simulink model "fuzzyReg_v10"  (R2022b)
settings: Solver=ode45  StartTime=0.0  StopTime=4  RelTol=1e-6  EnableMultiTasking=on
model workspace (MAT data in the model file):
  fuzzy33_v2 : mamfis (value not decoded)
  fuzzy55 : mamfis (value not decoded)
  fuzzy55_v2 : mamfis (value not decoded)
undefined symbols (not defined in the file or in its folder): Cfi, Imax, J, Jc, Ka, KI, KR, KRw, KTM, Kw, Mz, sigbuilder_block, Ta, TI, TIw, TTM, Un, w0
libraries: fuzblock x4
settings Model: Creator=Samuel  LastModifiedBy=hwswi
settings SolverCC: AlgebraicLoopSolver=TrustRegion
settings DataIOCC: LimitDataPoints=on  SaveFormat=Array  ReturnWorkspaceOutputs=off
settings OptimizationCC: LifeSpan=inf
settings DebuggingCC: UnconnectedInputMsg=warning  UnconnectedOutputMsg=warning  UnconnectedLineMsg=warning  SFUnexpectedBacktrackingDiag=warning  SFNoUnconditionalDefaultTransitionDiag=warning  SFExecutionAtInitializationDiag=none  SFMachineParentedDataDiag=warning  ArithmeticOperatorsInVariantConditions=warning
settings HardwareCC: ProdBitPerPointer=32  ProdBitPerSizeT=32  ProdBitPerPtrDiffT=32  ProdLargestAtomicFloat=None  ProdIntDivRoundTo=Undefined  ProdEndianess=Unspecified  ProdWordSize=32  ProdHWDeviceType=32-bit Generic
settings ModelReferenceCC: PropagateSignalLabelsOutOfModel=off
settings SFSimCC: SimUseLocalCustomCode=off  CustomCodeUndefinedFunction=UseInterfaceOnly
settings RTWCC: RTWUseLocalCustomCode=off
settings CodeAppCC: StateflowObjectComments=on
settings GRTTargetCC: TargetLangStandard=C89/C90 (ANSI)
settings ConfigComp: CovMetricSettings=dw  CovSaveCumulativeToWorkspaceVar=on  CovSaveSingleToWorkspaceVar=on  CovExternalEMLEnable=off

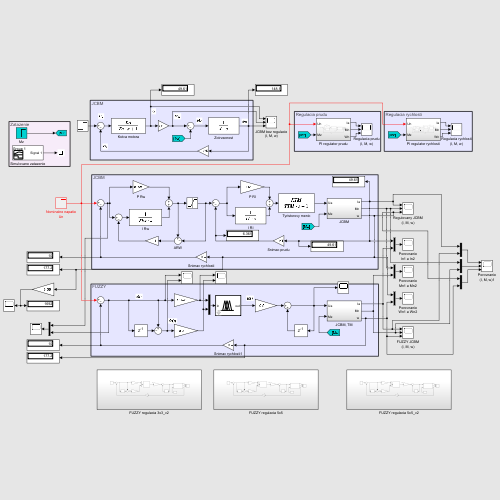
[thumbnail: Simulink's stored preview of the top-level diagram]
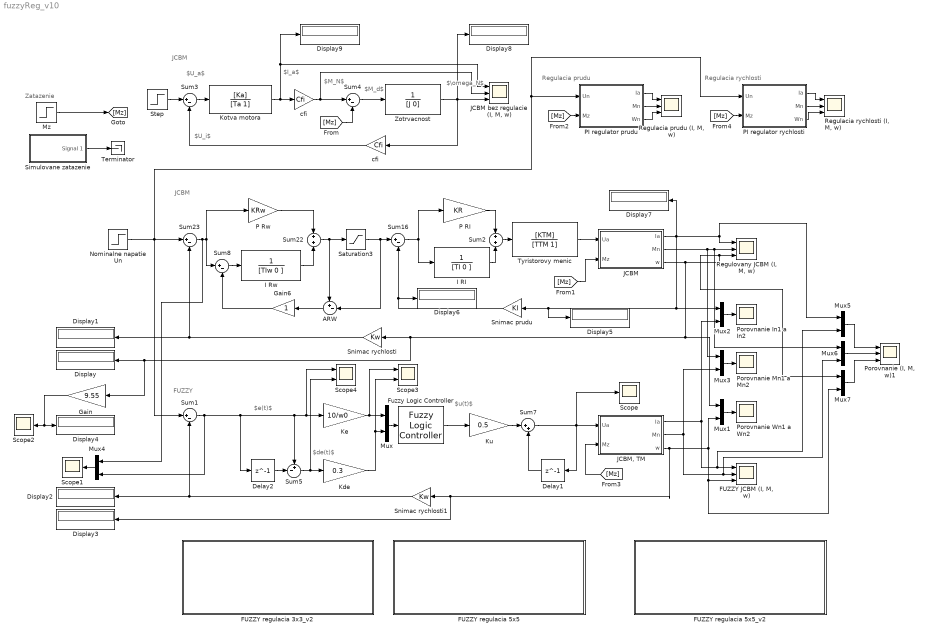
== system fuzzyReg_v10 ==
  note: Regulacia prudu
  note: Zatazenie
  note: JCBM
  note: FUZZY
  note: JCBM
  note: $M_N$
  note: $M_d$
  note: $I_a$
  note: $U_a$
  note: $U_i$
  note: $\omega_N$
  note: $e(t)$
  note: $de(t)$
  note: $u(t)$
  note: Regulacia rychlosti
  ARW : Sum  Inputs=+-|
  Delay1 : Delay  DelayLength=1  InitialCondition=0  SampleTime=0.018
  Delay2 : Delay  DelayLength=1  InitialCondition=0  SampleTime=0.018
  Display{,1..9} (10 alike) : Display
  "FUZZY JCBM (I, M, w)" : Scope  NumInputPorts=3
  FUZZY regulacia 3x3_v2 : Subsystem
  FUZZY regulacia 5x5 : Subsystem
  FUZZY regulacia 5x5_v2 : Subsystem
  Fuzzy Logic Controller : fuzblock/Fuzzy Logic  Controller  FIS=fuzzy55_v2  OutputSampleNumber=101  DataType=double  FuzzifiedInputs=off  RuleFiringStrengths=off  RuleOutputs=off  AggregatedOutputs=off  SimulateUsing=Interpreted execution  OutOfRangeInputValueMessage=warning  NoRuleFiredMessage=warning  EmptyOutputFuzzySetMessage=warning
  Gain : Gain  Gain=9.55
  Gain6 : Gain
  I RI : TransferFcn  Denominator=[TI 0 ]
  I Rw : TransferFcn  Denominator=[TIw 0 ]
  JCBM : Subsystem
  "JCBM bez regulacie (I, M, w)" : Scope  NumInputPorts=3
  "JCBM, TM" : Subsystem
  Kde : Gain  Gain=0.3
  Ke : Gain  Gain=10/w0
  Kotva motora : TransferFcn  Numerator=[Ka]  Denominator=[Ta 1]
  Ku : Gain  Gain=0.5
  Mux{,1..7} (8 alike) : Mux  Inputs=2
  Mz : Step  Time=2  After=Mz  SampleTime=0
  Nominalne napatie Un : Step  Time=0  After=10  SampleTime=0
  P RI : Gain  Gain=KR
  P Rw : Gain  Gain=KRw
  PI regulator prudu : Subsystem
  PI regulator rychlosti : Subsystem
  "Porovnanie (I, M, w)1" : Scope  NumInputPorts=3
  Porovnanie In1 a In2 : Scope
  Porovnanie Mn1 a Mn2 : Scope
  Porovnanie Wn1 a Wn2 : Scope
  "Regulacia prudu (I, M, w)" : Scope  NumInputPorts=3
  "Regulacia rychlosti (I, M, w)" : Scope  NumInputPorts=3
  "Regulovany JCBM (I, M, w)" : Scope  NumInputPorts=3
  Saturation3 : Saturate  UpperLimit=10  LowerLimit=-10
  Scope : Scope
  Scope1 : Scope
  Scope2 : Scope
  Scope3 : Scope  NumInputPorts=2
  Scope4 : Scope  NumInputPorts=2
  Simulovane zatazenie : Subsystem  Tag=STV Subsys  LoadFcn=sigbuilder_block('load');  StartFcn=sigbuilder_block('start');  StopFcn=sigbuilder_block('stop');  ClipboardFcn=sigbuilder_block('clipboard');  mask(Sigbuilder block){tuvar=[0:10]}
      mask help: Simulink:masks:SigbuilderBlock_MD
      mask init:
      | if ~strcmp(get_param(bdroot(gcbh),'SimulationStatus'),'stopped') tuvar = sigbuilder_block('maskInit'); end
      settings: CopyFcn=sigbuilder_block('copy');  DeleteFcn=sigbuilder_block('delete');  ModelCloseFcn=sigbuilder_block('modelClose');  PreSaveFcn=sigbuilder_block('preSave');  PauseFcn=sigbuilder_block('pause');  ContinueFcn=sigbuilder_block('continue');  NameChangeFcn=sigbuilder_block('namechange');  OpenFcn=sigbuilder_block('open',[717 162.75 551.25 360 ]);  CloseFcn=sigbuilder_block('close');
      mask Display: plot(0, 0, 100, 100,[2, 2, 32, 32, 2], [68, 8, 8, 68, 68],[32, 2], [38, 38], [32, 19, 2],[53, 60, 44], [32, 17, 17, 2],[16, 16, 31, 31]);txt = getActiveGroup(gcbh);text(2, 100, txt,'verticalAlignment', 'top');
  Snimac prudu : Gain  Gain=KI
  Snimac rychlosti : Gain  Gain=Kw
  Snimac rychlosti1 : Gain  Gain=Kw
  Step : Step  Time=0  After=Un  SampleTime=0
  Sum{1,3..4,8,16,23} (6 alike) : Sum  Inputs=|+-
  Sum2 : Sum
  Sum22 : Sum
  Sum5 : Sum  Inputs=+-|
  Sum7 : Sum  Inputs=|++
  Terminator : Terminator
  Tyristorovy menic : TransferFcn  Numerator=[KTM]  Denominator=[TTM 1]
  Zotrvacnost : TransferFcn  Denominator=[J 0]
  cfi : Gain  Gain=Cfi
  "cfi " : Gain  Gain=Cfi
  wires:
  Mux1/1 -> Porovnanie Wn1 a Wn2/1
  Mux2/1 -> Porovnanie In1 a In2/1
  Gain6/1 -> Sum8/2
  Sum8/1 -> I Rw/1
  ARW/1 -> Gain6/1
  Snimac rychlosti/1 -> Sum23/2, Display1/1
  Sum22/1 -> Saturation3/1, ARW/1
  I Rw/1 -> Sum22/2
  P Rw/1 -> Sum22/1
  Tyristorovy menic/1 -> JCBM/1(Ua)
  Sum23/1 -> Sum8/1, P Rw/1, Mux4/1
  Snimac prudu/1 -> Display6/1, Sum16/2
  Saturation3/1 -> ARW/2, Sum16/1
  Sum16/1 -> I RI/1, P RI/1
  Sum2/1 -> Tyristorovy menic/1
  I RI/1 -> Sum2/2
  P RI/1 -> Sum2/1
  JCBM/1(Ia) -> Display7/1, Mux5/1, "Regulovany JCBM (I, M, w)"/1, Mux2/1, Display5/1, Snimac prudu/1
  "JCBM, TM"/1(Ia) -> Mux2/2, Mux5/2, "FUZZY JCBM (I, M, w)"/1
  Sum5/1 -> Kde/1, Scope4/2
  Kde/1 -> Scope3/2, Mux/2
  Delay1/1 -> Sum7/2
  Delay2/1 -> Sum5/2
  Ke/1 -> Scope3/1, Mux/1
  Sum7/1 -> Delay1/1, Scope/1, "JCBM, TM"/1(Ua)
  Ku/1 -> Sum7/1
  Zotrvacnost/1 -> Display8/1, "JCBM bez regulacie (I, M, w)"/3, cfi/1
  cfi/1 -> Sum3/2
  Sum4/1 -> Zotrvacnost/1
  "cfi "/1 -> "JCBM bez regulacie (I, M, w)"/2, Sum4/1
  Sum3/1 -> Kotva motora/1
  [Mz] -> Sum4/2
  Mz/1 -> [Mz]
  [Mz] -> JCBM/2(Mz)
  PI regulator prudu/2(Mn) -> "Regulacia prudu (I, M, w)"/2
  PI regulator prudu/1(Ia) -> "Regulacia prudu (I, M, w)"/1
  PI regulator prudu/3(Wn) -> "Regulacia prudu (I, M, w)"/3
  [Mz] -> PI regulator prudu/2(Mz)
  "JCBM, TM"/2(" Mn ") -> Mux3/2, "FUZZY JCBM (I, M, w)"/2, Mux6/2
  JCBM/2(" Mn ") -> Mux3/1, "Regulovany JCBM (I, M, w)"/2, Mux6/1
  Mux3/1 -> Porovnanie Mn1 a Mn2/1
  Mux/1 -> Fuzzy Logic Controller/1
  Fuzzy Logic Controller/1 -> Ku/1
  [Mz] -> "JCBM, TM"/2(Mz)
  JCBM/3("w ") -> Mux7/1, "Regulovany JCBM (I, M, w)"/3, Mux1/1, Gain/1, Display/1, Snimac rychlosti/1
  Mux5/1 -> "Porovnanie (I, M, w)1"/1
  Mux6/1 -> "Porovnanie (I, M, w)1"/2
  Mux7/1 -> "Porovnanie (I, M, w)1"/3
  Snimac rychlosti1/1 -> Sum1/2, Display2/1
  Mux4/1 -> Scope1/1
  Gain/1 -> Scope2/1, Display4/1
  Sum1/1 -> Delay2/1, Ke/1, Scope4/1, Sum5/1, Mux4/2
  "JCBM, TM"/3("w ") -> Display3/1, Snimac rychlosti1/1, "FUZZY JCBM (I, M, w)"/3, Mux7/2, Mux1/2
  Nominalne napatie Un/1 -> Sum23/1, Sum1/1, PI regulator rychlosti/1(Un), PI regulator prudu/1(Un)
  Kotva motora/1 -> Display9/1, "JCBM bez regulacie (I, M, w)"/1, "cfi "/1
  Step/1 -> Sum3/1
  [Mz] -> PI regulator rychlosti/2(Mz)
  PI regulator rychlosti/3(Wn) -> "Regulacia rychlosti (I, M, w)"/3
  PI regulator rychlosti/1(Ia) -> "Regulacia rychlosti (I, M, w)"/1
  PI regulator rychlosti/2(Mn) -> "Regulacia rychlosti (I, M, w)"/2
  Simulovane zatazenie/1(Signal 1) -> Terminator/1

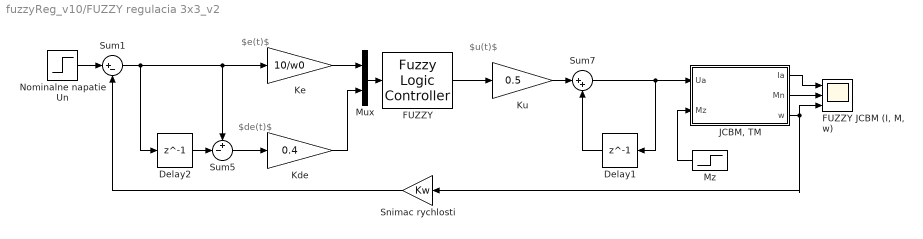
== system fuzzyReg_v10/FUZZY regulacia 3x3_v2 ==
  note: $e(t)$
  note: $de(t)$
  note: $u(t)$
  Delay1 : Delay  DelayLength=1  InitialCondition=0  SampleTime=0.018
  Delay2 : Delay  DelayLength=1  InitialCondition=0  SampleTime=0.018
  FUZZY : fuzblock/Fuzzy Logic  Controller  FIS=fuzzy33_v2  OutputSampleNumber=101  DataType=double  FuzzifiedInputs=off  RuleFiringStrengths=off  RuleOutputs=off  AggregatedOutputs=off  SimulateUsing=Interpreted execution  OutOfRangeInputValueMessage=warning  NoRuleFiredMessage=warning  EmptyOutputFuzzySetMessage=warning
  "FUZZY JCBM (I, M, w)" : Scope  NumInputPorts=3
  "JCBM, TM" : Subsystem
  Kde : Gain  Gain=0.4
  Ke : Gain  Gain=10/w0
  Ku : Gain  Gain=0.5
  Mux : Mux  Inputs=2
  Mz : Step  Time=2  After=Mz  SampleTime=0
  Nominalne napatie Un : Step  Time=0  After=10  SampleTime=0
  Snimac rychlosti : Gain  Gain=Kw
  Sum1 : Sum  Inputs=|+-
  Sum5 : Sum  Inputs=+-|
  Sum7 : Sum  Inputs=|++
  wires:
  Mz/1 -> "JCBM, TM"/2(Mz)
  Sum5/1 -> Kde/1
  Kde/1 -> Mux/2
  Sum1/1 -> Delay2/1, Ke/1, Sum5/1
  "JCBM, TM"/2(" Mn ") -> "FUZZY JCBM (I, M, w)"/2
  Sum7/1 -> Delay1/1, "JCBM, TM"/1(Ua)
  Ku/1 -> Sum7/1
  "JCBM, TM"/1(Ia) -> "FUZZY JCBM (I, M, w)"/1
  Ke/1 -> Mux/1
  Mux/1 -> FUZZY/1
  Nominalne napatie Un/1 -> Sum1/1
  Snimac rychlosti/1 -> Sum1/2
  "JCBM, TM"/3("w ") -> Snimac rychlosti/1, "FUZZY JCBM (I, M, w)"/3
  Delay1/1 -> Sum7/2
  FUZZY/1 -> Ku/1
  Delay2/1 -> Sum5/2

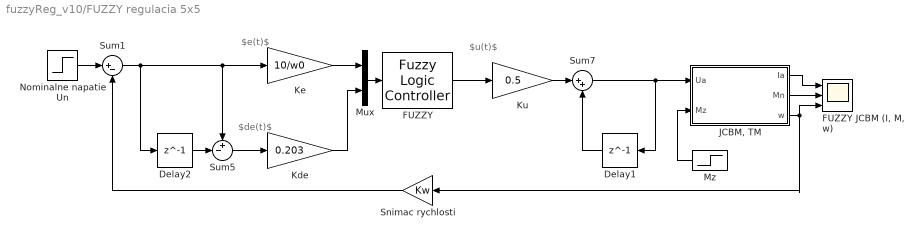
== system fuzzyReg_v10/FUZZY regulacia 5x5 ==
  note: $e(t)$
  note: $de(t)$
  note: $u(t)$
  Delay1 : Delay  DelayLength=1  InitialCondition=0  SampleTime=0.018
  Delay2 : Delay  DelayLength=1  InitialCondition=0  SampleTime=0.018
  FUZZY : fuzblock/Fuzzy Logic  Controller  FIS=fuzzy33_v2  OutputSampleNumber=101  DataType=double  FuzzifiedInputs=off  RuleFiringStrengths=off  RuleOutputs=off  AggregatedOutputs=off  SimulateUsing=Interpreted execution  OutOfRangeInputValueMessage=warning  NoRuleFiredMessage=warning  EmptyOutputFuzzySetMessage=warning
  "FUZZY JCBM (I, M, w)" : Scope  NumInputPorts=3
  "JCBM, TM" : Subsystem
  Kde : Gain  Gain=0.203
  Ke : Gain  Gain=10/w0
  Ku : Gain  Gain=0.5
  Mux : Mux  Inputs=2
  Mz : Step  Time=2  After=Mz  SampleTime=0
  Nominalne napatie Un : Step  Time=0  After=10  SampleTime=0
  Snimac rychlosti : Gain  Gain=Kw
  Sum1 : Sum  Inputs=|+-
  Sum5 : Sum  Inputs=+-|
  Sum7 : Sum  Inputs=|++
  wires:
  Mz/1 -> "JCBM, TM"/2(Mz)
  Sum5/1 -> Kde/1
  Kde/1 -> Mux/2
  Sum1/1 -> Delay2/1, Ke/1, Sum5/1
  "JCBM, TM"/2(" Mn ") -> "FUZZY JCBM (I, M, w)"/2
  Sum7/1 -> Delay1/1, "JCBM, TM"/1(Ua)
  Ku/1 -> Sum7/1
  "JCBM, TM"/1(Ia) -> "FUZZY JCBM (I, M, w)"/1
  Ke/1 -> Mux/1
  Mux/1 -> FUZZY/1
  Nominalne napatie Un/1 -> Sum1/1
  Snimac rychlosti/1 -> Sum1/2
  "JCBM, TM"/3("w ") -> Snimac rychlosti/1, "FUZZY JCBM (I, M, w)"/3
  Delay1/1 -> Sum7/2
  FUZZY/1 -> Ku/1
  Delay2/1 -> Sum5/2

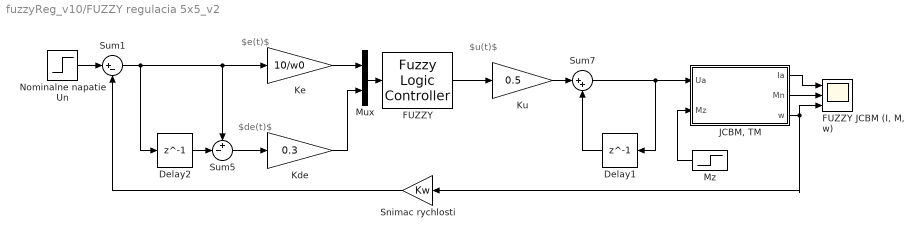
== system fuzzyReg_v10/FUZZY regulacia 5x5_v2 ==
  note: $u(t)$
  note: $de(t)$
  note: $e(t)$
  Delay1 : Delay  DelayLength=1  InitialCondition=0  SampleTime=0.018
  Delay2 : Delay  DelayLength=1  InitialCondition=0  SampleTime=0.018
  FUZZY : fuzblock/Fuzzy Logic  Controller  FIS=fuzzy33_v2  OutputSampleNumber=101  DataType=double  FuzzifiedInputs=off  RuleFiringStrengths=off  RuleOutputs=off  AggregatedOutputs=off  SimulateUsing=Interpreted execution  OutOfRangeInputValueMessage=warning  NoRuleFiredMessage=warning  EmptyOutputFuzzySetMessage=warning
  "FUZZY JCBM (I, M, w)" : Scope  NumInputPorts=3
  "JCBM, TM" : Subsystem
  Kde : Gain  Gain=0.3
  Ke : Gain  Gain=10/w0
  Ku : Gain  Gain=0.5
  Mux : Mux  Inputs=2
  Mz : Step  Time=2  After=Mz  SampleTime=0
  Nominalne napatie Un : Step  Time=0  After=10  SampleTime=0
  Snimac rychlosti : Gain  Gain=Kw
  Sum1 : Sum  Inputs=|+-
  Sum5 : Sum  Inputs=+-|
  Sum7 : Sum  Inputs=|++
  wires:
  Delay2/1 -> Sum5/2
  FUZZY/1 -> Ku/1
  Delay1/1 -> Sum7/2
  "JCBM, TM"/3("w ") -> "FUZZY JCBM (I, M, w)"/3, Snimac rychlosti/1
  Snimac rychlosti/1 -> Sum1/2
  Nominalne napatie Un/1 -> Sum1/1
  Mux/1 -> FUZZY/1
  Ke/1 -> Mux/1
  "JCBM, TM"/1(Ia) -> "FUZZY JCBM (I, M, w)"/1
  Ku/1 -> Sum7/1
  Sum7/1 -> "JCBM, TM"/1(Ua), Delay1/1
  "JCBM, TM"/2(" Mn ") -> "FUZZY JCBM (I, M, w)"/2
  Sum1/1 -> Sum5/1, Ke/1, Delay2/1
  Kde/1 -> Mux/2
  Sum5/1 -> Kde/1
  Mz/1 -> "JCBM, TM"/2(Mz)

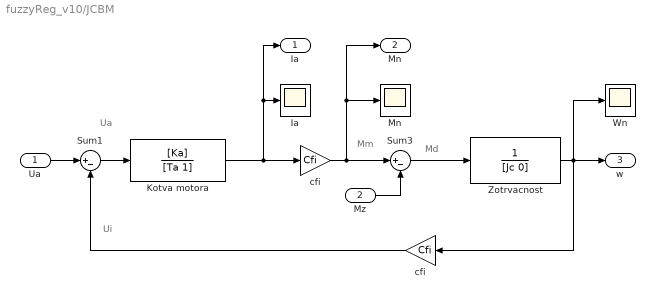
== system fuzzyReg_v10/JCBM ==
  note: Ui
  note: Ua
  note: Mm
  note: Md
  Ua : Inport
  Mz : Inport  Port=2
  "Ia " : Scope
  Kotva motora : TransferFcn  Numerator=[Ka]  Denominator=[Ta 1]
  "Mn " : Scope
  Sum1 : Sum  Inputs=|+-
  Sum3 : Sum  Inputs=|+-
  Wn : Scope
  Zotrvacnost : TransferFcn  Denominator=[Jc 0]
  cfi : Gain  Gain=Cfi
  "cfi " : Gain  Gain=Cfi
  Ia : Outport
  " Mn " : Outport  Port=2
  "w " : Outport  Port=3
  wires:
  Sum1/1 -> Kotva motora/1
  Mz/1 -> Sum3/2
  Zotrvacnost/1 -> Wn/1, "w "/1, cfi/1
  Ua/1 -> Sum1/1
  cfi/1 -> Sum1/2
  "cfi "/1 -> " Mn "/1, "Mn "/1, Sum3/1
  Kotva motora/1 -> "cfi "/1, Ia/1, "Ia "/1
  Sum3/1 -> Zotrvacnost/1

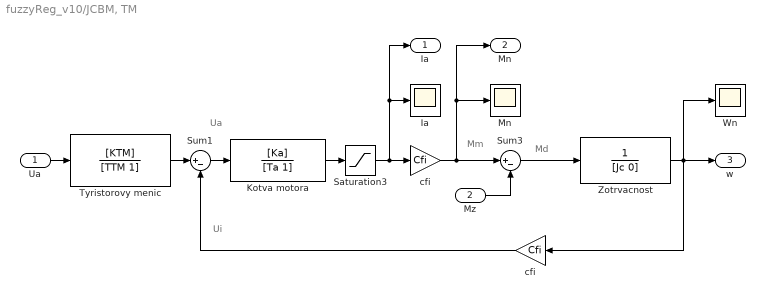
== system fuzzyReg_v10/JCBM, TM ==
  note: Ui
  note: Ua
  note: Mm
  note: Md
  Ua : Inport
  Mz : Inport  Port=2
  "Ia " : Scope
  Kotva motora : TransferFcn  Numerator=[Ka]  Denominator=[Ta 1]
  "Mn " : Scope
  Saturation3 : Saturate  UpperLimit=Imax  LowerLimit=-Imax
  Sum1 : Sum  Inputs=|+-
  Sum3 : Sum  Inputs=|+-
  Tyristorovy menic : TransferFcn  Numerator=[KTM]  Denominator=[TTM 1]
  Wn : Scope
  Zotrvacnost : TransferFcn  Denominator=[Jc 0]
  cfi : Gain  Gain=Cfi
  "cfi " : Gain  Gain=Cfi
  Ia : Outport
  " Mn " : Outport  Port=2
  "w " : Outport  Port=3
  wires:
  Sum1/1 -> Kotva motora/1
  Mz/1 -> Sum3/2
  Zotrvacnost/1 -> Wn/1, "w "/1, cfi/1
  Ua/1 -> Tyristorovy menic/1
  cfi/1 -> Sum1/2
  "cfi "/1 -> " Mn "/1, "Mn "/1, Sum3/1
  Sum3/1 -> Zotrvacnost/1
  Tyristorovy menic/1 -> Sum1/1
  Kotva motora/1 -> Saturation3/1
  Saturation3/1 -> Ia/1, "Ia "/1, "cfi "/1

== system fuzzyReg_v10/PI regulator prudu ==
  Un : Inport
  Mz : Inport  Port=2
  I : TransferFcn  Denominator=[TI 0 ]
  JCBM : Subsystem
  P : Gain  Gain=KR
  Snimac prudu : Gain  Gain=KI
  Sum16 : Sum  Inputs=|+-
  Sum2 : Sum
  Tyristorovy menic : TransferFcn  Numerator=[KTM]  Denominator=[TTM 1]
  Ia : Outport
  Mn : Outport  Port=2
  Wn : Outport  Port=3
  wires:
  Mz/1 -> JCBM/2(Mz)
  JCBM/2(" Mn ") -> Mn/1
  Tyristorovy menic/1 -> JCBM/1(Ua)
  Un/1 -> Sum16/1
  Sum2/1 -> Tyristorovy menic/1
  Snimac prudu/1 -> Sum16/2
  Sum16/1 -> I/1, P/1
  JCBM/1(Ia) -> Ia/1, Snimac prudu/1
  JCBM/3("w ") -> Wn/1
  I/1 -> Sum2/2
  P/1 -> Sum2/1

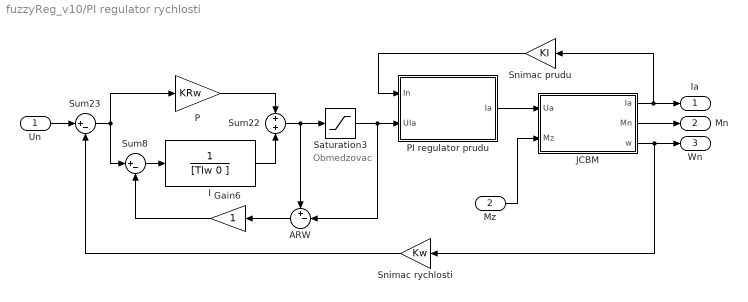
== system fuzzyReg_v10/PI regulator rychlosti ==
  note: Obmedzovac
  Un : Inport
  Mz : Inport  Port=2
  ARW : Sum  Inputs=+-|
  Gain6 : Gain
  I : TransferFcn  Denominator=[TIw 0 ]
  JCBM : Subsystem
  P : Gain  Gain=KRw
  PI regulator prudu : Subsystem
  Saturation3 : Saturate  UpperLimit=10  LowerLimit=-10
  Snimac prudu : Gain  Gain=KI
  Snimac rychlosti : Gain  Gain=Kw
  Sum22 : Sum
  Sum23 : Sum  Inputs=|+-
  Sum8 : Sum  Inputs=|+-
  Ia : Outport
  Mn : Outport  Port=2
  Wn : Outport  Port=3
  wires:
  Mz/1 -> JCBM/2(Mz)
  JCBM/2(" Mn ") -> Mn/1
  PI regulator prudu/1(Ia) -> JCBM/1(Ua)
  JCBM/1(Ia) -> Snimac prudu/1, Ia/1
  JCBM/3("w ") -> Snimac rychlosti/1, Wn/1
  Un/1 -> Sum23/1
  Sum8/1 -> I/1
  P/1 -> Sum22/1
  Saturation3/1 -> ARW/2, PI regulator prudu/2(UIa)
  ARW/1 -> Gain6/1
  Gain6/1 -> Sum8/2
  Sum23/1 -> Sum8/1, P/1
  I/1 -> Sum22/2
  Sum22/1 -> Saturation3/1, ARW/1
  Snimac rychlosti/1 -> Sum23/2
  Snimac prudu/1 -> PI regulator prudu/1(In)

== system fuzzyReg_v10/Simulovane zatazenie ==
  Demux : Demux  Tag=STV Demux  Outputs=1
      settings: DisplayOption=none
  FromWs : FromWorkspace  Tag=STV FromWs  VariableName=tuvar
      SigBuilderData=|
      | common.afterFinalStr = 'Extrapolate'
      | common.sampleTime = 0
      | dataSet.timeRange = [0 10]
      | dataSet.name = 'Group 1'
      | sbobj.Groups.Name = 'Group 1'
      | sbobj.Groups.Signals.Name = 'Signal 1'
      | sbobj.Groups.Signals.XData = [0 2 2 4 4 6 6 10]
      | sbobj.Groups.Signals.YData = [0 0 85 85 170 170 0 0]
  Signal 1 : Outport  Tag=STV Outport
  wires:
  FromWs/1 -> Demux/1
  Demux/1 -> Signal 1/1

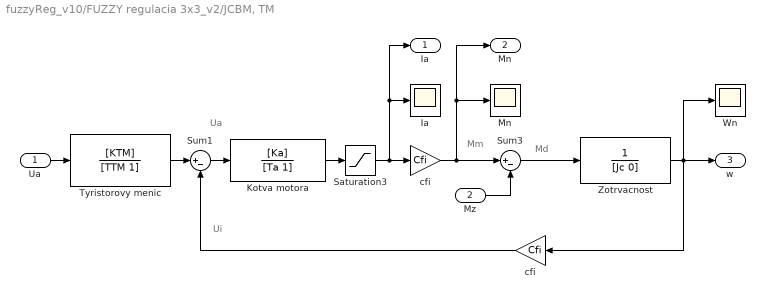
== system fuzzyReg_v10/FUZZY regulacia 3x3_v2/JCBM, TM ==
  note: Ui
  note: Ua
  note: Mm
  note: Md
  Ua : Inport
  Mz : Inport  Port=2
  "Ia " : Scope
  Kotva motora : TransferFcn  Numerator=[Ka]  Denominator=[Ta 1]
  "Mn " : Scope
  Saturation3 : Saturate  UpperLimit=Imax  LowerLimit=-Imax
  Sum1 : Sum  Inputs=|+-
  Sum3 : Sum  Inputs=|+-
  Tyristorovy menic : TransferFcn  Numerator=[KTM]  Denominator=[TTM 1]
  Wn : Scope
  Zotrvacnost : TransferFcn  Denominator=[Jc 0]
  cfi : Gain  Gain=Cfi
  "cfi " : Gain  Gain=Cfi
  Ia : Outport
  " Mn " : Outport  Port=2
  "w " : Outport  Port=3
  wires:
  Sum1/1 -> Kotva motora/1
  Mz/1 -> Sum3/2
  Zotrvacnost/1 -> Wn/1, "w "/1, cfi/1
  Ua/1 -> Tyristorovy menic/1
  cfi/1 -> Sum1/2
  "cfi "/1 -> " Mn "/1, "Mn "/1, Sum3/1
  Sum3/1 -> Zotrvacnost/1
  Tyristorovy menic/1 -> Sum1/1
  Kotva motora/1 -> Saturation3/1
  Saturation3/1 -> Ia/1, "Ia "/1, "cfi "/1

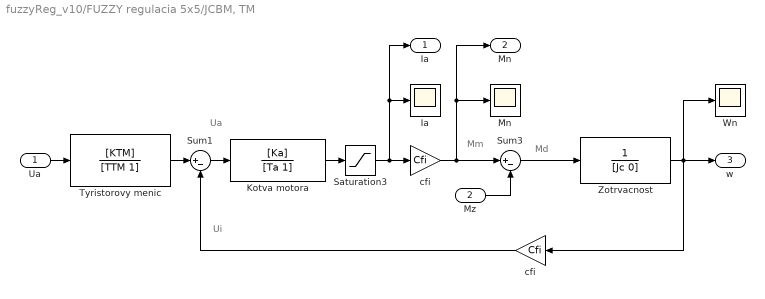
== system fuzzyReg_v10/FUZZY regulacia 5x5/JCBM, TM ==
  note: Ui
  note: Ua
  note: Mm
  note: Md
  Ua : Inport
  Mz : Inport  Port=2
  "Ia " : Scope
  Kotva motora : TransferFcn  Numerator=[Ka]  Denominator=[Ta 1]
  "Mn " : Scope
  Saturation3 : Saturate  UpperLimit=Imax  LowerLimit=-Imax
  Sum1 : Sum  Inputs=|+-
  Sum3 : Sum  Inputs=|+-
  Tyristorovy menic : TransferFcn  Numerator=[KTM]  Denominator=[TTM 1]
  Wn : Scope
  Zotrvacnost : TransferFcn  Denominator=[Jc 0]
  cfi : Gain  Gain=Cfi
  "cfi " : Gain  Gain=Cfi
  Ia : Outport
  " Mn " : Outport  Port=2
  "w " : Outport  Port=3
  wires:
  Sum1/1 -> Kotva motora/1
  Mz/1 -> Sum3/2
  Zotrvacnost/1 -> Wn/1, "w "/1, cfi/1
  Ua/1 -> Tyristorovy menic/1
  cfi/1 -> Sum1/2
  "cfi "/1 -> " Mn "/1, "Mn "/1, Sum3/1
  Sum3/1 -> Zotrvacnost/1
  Tyristorovy menic/1 -> Sum1/1
  Kotva motora/1 -> Saturation3/1
  Saturation3/1 -> Ia/1, "Ia "/1, "cfi "/1

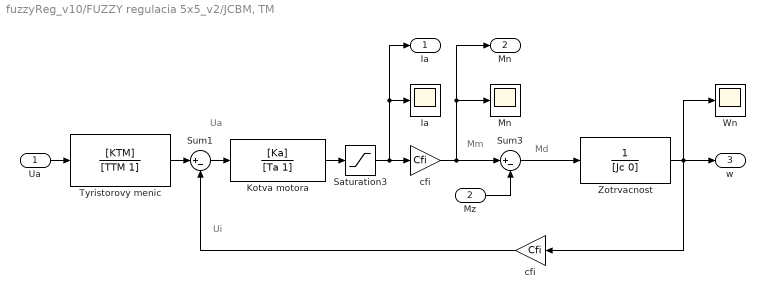
== system fuzzyReg_v10/FUZZY regulacia 5x5_v2/JCBM, TM ==
  note: Md
  note: Mm
  note: Ua
  note: Ui
  Ua : Inport
  Mz : Inport  Port=2
  "Ia " : Scope
  Kotva motora : TransferFcn  Numerator=[Ka]  Denominator=[Ta 1]
  "Mn " : Scope
  Saturation3 : Saturate  UpperLimit=Imax  LowerLimit=-Imax
  Sum1 : Sum  Inputs=|+-
  Sum3 : Sum  Inputs=|+-
  Tyristorovy menic : TransferFcn  Numerator=[KTM]  Denominator=[TTM 1]
  Wn : Scope
  Zotrvacnost : TransferFcn  Denominator=[Jc 0]
  cfi : Gain  Gain=Cfi
  "cfi " : Gain  Gain=Cfi
  Ia : Outport
  " Mn " : Outport  Port=2
  "w " : Outport  Port=3
  wires:
  Saturation3/1 -> "cfi "/1, "Ia "/1, Ia/1
  Kotva motora/1 -> Saturation3/1
  Tyristorovy menic/1 -> Sum1/1
  Sum3/1 -> Zotrvacnost/1
  "cfi "/1 -> Sum3/1, "Mn "/1, " Mn "/1
  cfi/1 -> Sum1/2
  Ua/1 -> Tyristorovy menic/1
  Zotrvacnost/1 -> cfi/1, "w "/1, Wn/1
  Mz/1 -> Sum3/2
  Sum1/1 -> Kotva motora/1

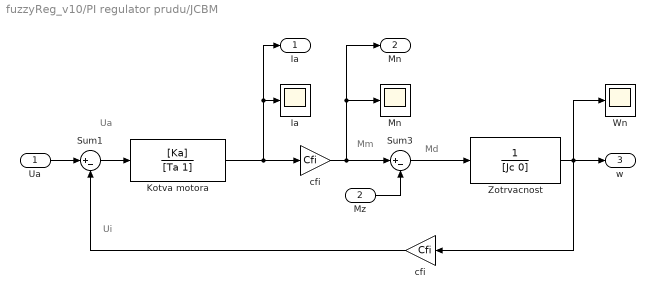
== system fuzzyReg_v10/PI regulator prudu/JCBM ==
  note: Ui
  note: Ua
  note: Mm
  note: Md
  Ua : Inport
  Mz : Inport  Port=2
  "Ia " : Scope
  Kotva motora : TransferFcn  Numerator=[Ka]  Denominator=[Ta 1]
  "Mn " : Scope
  Sum1 : Sum  Inputs=|+-
  Sum3 : Sum  Inputs=|+-
  Wn : Scope
  Zotrvacnost : TransferFcn  Denominator=[Jc 0]
  cfi : Gain  Gain=Cfi
  "cfi " : Gain  Gain=Cfi
  Ia : Outport
  " Mn " : Outport  Port=2
  "w " : Outport  Port=3
  wires:
  Sum1/1 -> Kotva motora/1
  Mz/1 -> Sum3/2
  Zotrvacnost/1 -> Wn/1, "w "/1, cfi/1
  Ua/1 -> Sum1/1
  cfi/1 -> Sum1/2
  "cfi "/1 -> " Mn "/1, "Mn "/1, Sum3/1
  Kotva motora/1 -> "cfi "/1, Ia/1, "Ia "/1
  Sum3/1 -> Zotrvacnost/1

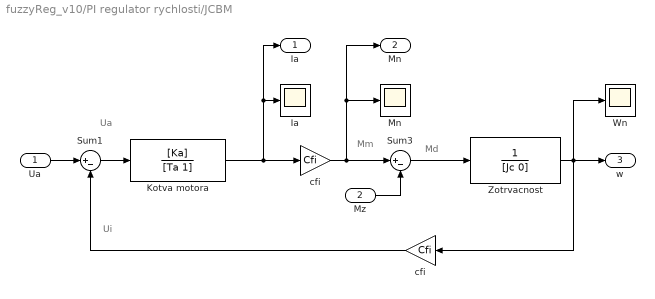
== system fuzzyReg_v10/PI regulator rychlosti/JCBM ==
  note: Ui
  note: Ua
  note: Mm
  note: Md
  Ua : Inport
  Mz : Inport  Port=2
  "Ia " : Scope
  Kotva motora : TransferFcn  Numerator=[Ka]  Denominator=[Ta 1]
  "Mn " : Scope
  Sum1 : Sum  Inputs=|+-
  Sum3 : Sum  Inputs=|+-
  Wn : Scope
  Zotrvacnost : TransferFcn  Denominator=[Jc 0]
  cfi : Gain  Gain=Cfi
  "cfi " : Gain  Gain=Cfi
  Ia : Outport
  " Mn " : Outport  Port=2
  "w " : Outport  Port=3
  wires:
  Sum1/1 -> Kotva motora/1
  Mz/1 -> Sum3/2
  Zotrvacnost/1 -> Wn/1, "w "/1, cfi/1
  Ua/1 -> Sum1/1
  cfi/1 -> Sum1/2
  "cfi "/1 -> " Mn "/1, "Mn "/1, Sum3/1
  Kotva motora/1 -> "cfi "/1, Ia/1, "Ia "/1
  Sum3/1 -> Zotrvacnost/1

== system fuzzyReg_v10/PI regulator rychlosti/PI regulator prudu ==
  In : Inport
  UIa : Inport  Port=2
  I : TransferFcn  Denominator=[TI 0 ]
  P : Gain  Gain=KR
  Sum16 : Sum  Inputs=|+-
  Sum2 : Sum
  Tyristorovy menic : TransferFcn  Numerator=[KTM]  Denominator=[TTM 1]
  Ia : Outport
  wires:
  Tyristorovy menic/1 -> Ia/1
  UIa/1 -> Sum16/1
  Sum2/1 -> Tyristorovy menic/1
  Sum16/1 -> I/1, P/1
  I/1 -> Sum2/2
  P/1 -> Sum2/1
  In/1 -> Sum16/2
